simulink model "drone_sim_2"  (R2022b)
settings: Solver=VariableStepAuto  StartTime=0.0  StopTime=10.0  RelTol=1e-3
values from neighbouring files (symbols this model uses):
  m = 1    [drone_2.m]    (also in path_generation.m; pid_test.m; trajectory.m)
  p0 = [0;0;0]    [drone.m]    (also in drone_2.m)
  v0 = [0;0;0]    [drone.m]    (also in drone_2.m)
settings Model: Creator=simonecarena  LastModifiedBy=simonecarena

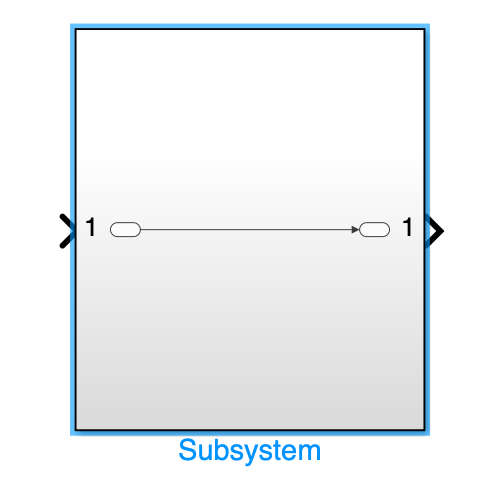
[thumbnail: Simulink's stored preview of the top-level diagram]
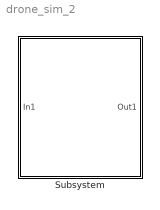
== system drone_sim_2 ==
  Subsystem : Subsystem

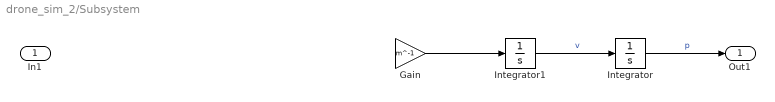
== system drone_sim_2/Subsystem ==
  In1 : Inport
  Gain : Gain  Gain=m^-1
  Integrator : Integrator  InitialCondition=p0
  Integrator1 : Integrator  InitialCondition=v0
  Out1 : Outport
  wires:
  Integrator/1 -> Out1/1  "p"
  Integrator1/1 -> Integrator/1  "v"
  Gain/1 -> Integrator1/1
